simulink model "Host Code"  (R2019b)
settings: Solver=FixedStepAuto  StartTime=0.0  StopTime=inf  FixedStep=1e-2  RelTol=1e-3  EnableMultiTasking=on
libraries: c2000scilib x3, demo_controls x1
settings Model: Creator=aancelle  LastModifiedBy=Fadik
settings SolverCC: AutoInsertRateTranBlk=on
settings DataIOCC: LimitDataPoints=on  SaveFormat=Array  SignalLoggingSaveFormat=ModelDataLogs  ReturnWorkspaceOutputs=off
settings OptimizationCC: BlockReduction=off  LifeSpan=1  EfficientTunableParamExpr=on
settings DebuggingCC: UnderspecifiedInitializationDetection=Classic  MergeDetectMultiDrivingBlocksExec=none  SolverPrmCheckMsg=warning  AllowSymbolicDim=off  SFUnexpectedBacktrackingDiag=warning  SFNoUnconditionalDefaultTransitionDiag=warning  SFExecutionAtInitializationDiag=none  ArithmeticOperatorsInVariantConditions=warning
settings HardwareCC: ProdBitPerPointer=32  ProdBitPerSizeT=32  ProdBitPerPtrDiffT=32  ProdLargestAtomicFloat=None  ProdIntDivRoundTo=Undefined  ProdEndianess=Unspecified  ProdWordSize=32  ProdHWDeviceType=32-bit Generic
settings ModelReferenceCC: PropagateSignalLabelsOutOfModel=off
settings SFSimCC: SimCustomSourceCode=C:\Users\Fadik\OneDrive\Documents\3rd Year Project\SIMULINK\TEST\test1.m  SimUseLocalCustomCode=off  SimAnalyzeCustomCode=on  MATLABDynamicMemAlloc=off  CustomCodeUndefinedFunction=UseInterfaceOnly
settings RTWCC: Description=Real-Time Workshop Embedded Coder  SystemTargetFile=ert.tlc  TemplateMakefile=ert_default_tmf  GenerateReport=on  RTWUseLocalCustomCode=off  IncludeHyperlinkInReport=on  LaunchReport=on  GenerateTraceInfo=on  GenerateTraceReport=on  GenerateTraceReportSl=on  GenerateTraceReportSf=on  GenerateTraceReportEml=on
settings CodeAppCC: IgnoreCustomStorageClasses=off  StateflowObjectComments=on  InternalIdentifier=Classic
settings ERTTargetCC: MultiwordLength=2048  GenerateSampleERTMain=on  ERTCustomFileTemplate=example_file_process.tlc  ConvertIfToSwitch=off  SuppressUnreachableDefaultCases=off
settings ConfigComp: CovMetricSettings=dw  CovHtmlReporting=on  CovSaveCumulativeToWorkspaceVar=on  CovSaveSingleToWorkspaceVar=on  CovExternalEMLEnable=off

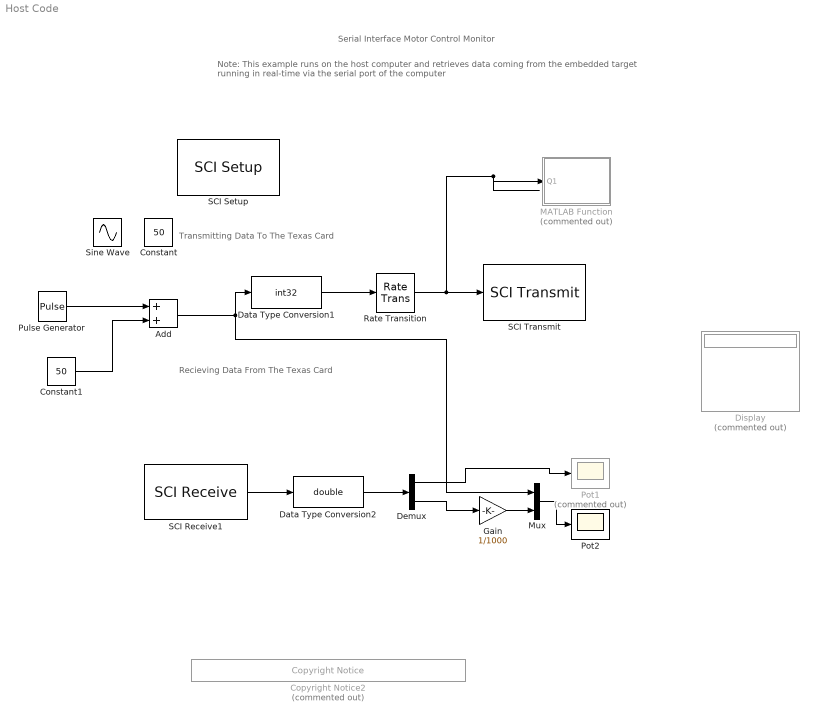
== system Host Code ==
  note: Transmitting Data To The Texas Card
  note: Note: This example runs on the host computer and retrieves data
      | coming from the embedded target running in real-time via the serial port of the computer
  note: Serial Interface Motor Control Monitor
  note: Recieving Data From The Texas Card
  Add : Sum
  Constant : Constant  Value=50
  Constant1 : Constant  Value=50
  Copyright Notice2 : demo_controls/Copyright Notice  Commented=on  year=2014  prod=tic2000
      settings: SourceProductName=MATLAB Coder  SourceProductBaseCode=ME
  Data Type Conversion1 : DataTypeConversion  OutDataTypeStr=int32  ConvertRealWorld=Stored Integer (SI)
  Data Type Conversion2 : DataTypeConversion  OutDataTypeStr=double
  Demux : Demux  Outputs=2
  Display : Display  Commented=on
  Gain : Gain  Gain=1/1000
  MATLAB Function : MATLAB Function  Commented=on  TreatAsAtomicUnit=on
  Mux : Mux  Inputs=2
  Pot1 : Scope  Commented=on
  Pot2 : Scope
  Pulse Generator : DiscretePulseGenerator  PulseType=Time based  Amplitude=50  Period=30  PulseWidth=50
  Rate Transition : RateTransition  OutPortSampleTime=0.1
  SCI Receive1 : c2000scilib/SCI Receive  module=COM 2  dataHead='S'  dataTail='E'  dataType=int32  dataDim=2  initValue=0  errOption=Output the last received value  errValue=0  sampleTime=0.1  outputStatus=off
      settings: SourceProductName=MATLAB Coder  SourceProductBaseCode=ME
  "SCI Setup " : c2000scilib/SCI Setup  Priority=-99  commModeA=raw data  baudRateA=115200  charLenA=8  stopBitA=1  parityA=none  timeoutA=1.0  commModeB=raw data  baudRateB=115200  charLenB=8  stopBitB=1  parityB=none  timeoutB=1.0  commModeC=raw data  baudRateC=115200  charLenC=8  stopBitC=1  parityC=none  timeoutC=1.0  commModeD=raw data  baudRateD=115200  charLenD=8  stopBitD=1  parityD=none  timeoutD=1.0
      settings: SourceProductName=MATLAB Coder  SourceProductBaseCode=ME
  SCI Transmit : c2000scilib/SCI Transmit  module=COM 2  header='S'  tail='E'
      settings: SourceProductName=MATLAB Coder  SourceProductBaseCode=ME
  Sine Wave : Sin  Amplitude=20  Bias=50  Frequency=0.01  SampleTime=0.1
  wires:
  Data Type Conversion1/1 -> Rate Transition/1
  Data Type Conversion2/1 -> Demux/1
  SCI Receive1/1 -> Data Type Conversion2/1
  Gain/1 -> Mux/2
  Demux/2 -> Gain/1
  Demux/1 -> Pot1/1
  Add/1 -> Data Type Conversion1/1, Mux/1
  Mux/1 -> Pot2/1
  Constant1/1 -> Add/2
  Pulse Generator/1 -> Add/1
  Rate Transition/1 -> MATLAB Function/1(Q1), SCI Transmit/1

== matlab function Host Code/MATLAB Function ==
  data: Q1 input
function fcn(Q1)
    
    %function h = ang(centre,radius,span,style)
        % ANG
        % Plots an angle arc with specified position and circumference.
        % Example:
        %                 ang([3 2],5,[0 pi/2],'k-')
        % Plots an arc with centre (3,2) and radius (5) that represents
        % The angle specified from 0 to pi/2, and with the preferred style 'k-'.
        % Draws heavily from Zhenhai Wang's circle function on the File Exchange.
        %
        % Husam Aldahiyat, October, 2008.

   %     theta = linspace(span(1),span(2),100);
   %     rho = ones(1,100) * radius;
   %     [x,y] = pol2cart(theta,rho);
    %    x = x + centre(1);
    %    y = y + centre(2);
    %    h = plot(x,y,style);
    %end

    q1v = [-pi/4,-pi/6, -pi/8, -pi/10, 0, pi/10, pi/8, pi/6, pi/4];
    q2v = [-pi/4,-pi/6, -pi/8, -pi/10, 0, pi/10, pi/8, pi/6, pi/4];
    l1 = 10; % length of first arm
    l2 = 10; % length of second arm
    pause(1.5);
    q1 = x;
    %input("What is Q1"); 
    %-pi/4;
    q2 = y;
    %input("What is Q2");
    %-pi/4;
    cla reset
    x1 = l1*cos(q1);
    x2 = l1*cos(q1) + l2*cos(q1+q2);
    x3 = l1*cos(q1) + l2*cos(q1);
    y1 = l1*sin(q1);
    y2 = l1*sin(q1) + l2*sin(q1+q2);
    y3 = l1*sin(q1) + l2*sin(q1);

    plot([0,x1],[0,y1],'b');
    xlim([-25,25]);
    ylim([-25,25]);
    hold on;
    plot([x1,x3],[y1,y3],'m--');
    plot([x1,x2],[y1,y2],'r');
    hold on;

   % ang([(0),(0)],1,[0,q1],'k-');
   % ang([(x1),(y1)],1,[q1,q1+q2],'k-');
end
